simulink model "Refined_Model_39"  (R2020b)
settings: Solver=FixedStepAuto  StartTime=0.0  StopTime=300  FixedStep=dt  RelTol=1e-3
values from neighbouring files (symbols this model uses):
  ALInpSpeed = AxlLoss (1,:)    [GPS_val.m]    (also in ICEBEV_Script.m; ICEBEV_Script_VECTO.m; ICE_Script.m; ICE_Script_SSVal.m)
  ALInpTor = AxlLoss(:,1)    [GPS_val.m]    (also in ICEBEV_Script.m; ICEBEV_Script_VECTO.m; ICE_Script.m; ICE_Script_SSVal.m)
  ALTableVal = AxlLoss(2:end,2:end)    [GPS_val.m]    (also in ICEBEV_Script.m; ICEBEV_Script_VECTO.m; ICE_Script.m; ICE_Script_SSVal.m)
  CovDist = RoadProfile(:,4)    [ICE_Val.m]
  Cx = VehicleDefine(7,3)    [BEV_Basictest.m]    (also in GPS_val.m; ICEBEV_Script.m; ICEBEV_Script_VECTO.m; ICE_Script.m)
  Dist = 1:length(MaxSpeedProfile)    [GPS_val.m]    (also in ICE_Script.m; ICE_Val.m = [1:CovDist(end)])
  DynRolRad = VehicleDefine(5,3)    [BEV_Basictest.m]    (also in GPS_val.m; ICEBEV_Script.m; ICEBEV_Script_VECTO.m; ICE_Script.m)
  EngineRpm = round(IntpTorCur(:,1))    [GPS_val.m]    (also in ICEBEV_Script.m; ICEBEV_Script_VECTO.m; ICE_Script.m; ICE_Script_SSVal.m)
  EngineRpmUse = [EngineRpmUse1; EngineRpmUse2]    [GPS_val.m]    (also in ICEBEV_Script.m; ICEBEV_Script_VECTO.m; ICE_Script.m; ICE_Script_SSVal.m)
  etaClutch = VehicleDefine(23,3)    [GPS_val.m]    (also in ICEBEV_Script.m; ICEBEV_Script_VECTO.m; ICE_Script.m; ICE_Script_SSVal.m)
  FCTableVal = FCMap(2:end,2:end)    [GPS_val.m]    (also in ICEBEV_Script.m; ICEBEV_Script_VECTO.m; ICE_Script.m; ICE_Script_SSVal.m)
  FDR = VehicleDefine(20,3)    [BEV_Basictest.m]    (also in GPS_val.m = VehicleDefine(22,3); ICEBEV_Script.m = VehicleDefine(22,3); ICEBEV_Script_VECTO.m = VehicleDefine(22,3); ICE_Script.m = VehicleDefine(22,3))
  Fr = VehicleDefine(13,3)    [BEV_Basictest.m]    (also in GPS_val.m; ICEBEV_Script.m; ICEBEV_Script_VECTO.m; ICE_Script.m)
  g = VehicleDefine(14,3)    [BEV_Basictest.m]    (also in GPS_val.m; ICEBEV_Script.m; ICEBEV_Script_VECTO.m; ICE_Script.m)
  GNo = GBXDefine(:,1)    [GPS_val.m]    (also in ICEBEV_Script.m; ICEBEV_Script_VECTO.m; ICE_Script.m; ICE_Script_SSVal.m)
  GRa = GBXDefine(:,2)    [GPS_val.m]    (also in ICEBEV_Script.m; ICEBEV_Script_VECTO.m; ICE_Script.m; ICE_Script_SSVal.m)
  InitVel = VehicleDefine(21,3)    [BEV_Basictest.m]    (also in GPS_val.m = VehicleDefine(24,3); ICEBEV_Script.m = VehicleDefine(24,3); ICEBEV_Script_VECTO.m = VehicleDefine(24,3); ICE_Script.m = VehicleDefine(24,3))
  IntpSlope = round(IntpSlope,1)    [GPS_val.m]    (also in ICE_Script.m; ICE_Val.m = A)
  Je = VehicleDefine(25,3)    [GPS_val.m]    (also in ICEBEV_Script.m; ICEBEV_Script_VECTO.m; ICE_Script.m; ICE_Script_SSVal.m)
  Jk = VehicleDefine(15,3)    [BEV_Basictest.m]    (also in GPS_val.m; ICEBEV_Script.m; ICEBEV_Script_VECTO.m; ICE_Script.m)
  Jm = VehicleDefine(16,3)    [GPS_val.m]    (also in ICEBEV_Script.m; ICEBEV_Script_VECTO.m; ICE_Script.m; ICE_Script_SSVal.m)
  MaxAcc = 1    [BEV_Basictest.m]    (also in GPS_val.m; ICEBEV_Script.m; ICEBEV_Script_VECTO.m; ICE_Script.m)
  MaxDec = 1    [BEV_Basictest.m]    (also in GPS_val.m; ICEBEV_Script.m; ICEBEV_Script_VECTO.m; ICE_Script.m)
  MaxSpeedProfile = FMSP    [GPS_val.m]    (also in ICE_Script.m; ICE_Val.m = repelem(SegSPLatinmps,SegLeninm))
  MaxTorValThrot = max(ThrotTableVal,[],2)    [GPS_val.m]    (also in ICEBEV_Script.m; ICEBEV_Script_VECTO.m; ICE_Script.m; ICE_Script_SSVal.m)
  Me = VehicleDefine(10,3)    [BEV_Basictest.m]    (also in GPS_val.m; ICEBEV_Script.m; ICEBEV_Script_VECTO.m; ICE_Script.m)
  MotoringTor = IntpTorCur(:,3)    [GPS_val.m]    (also in ICEBEV_Script.m; ICEBEV_Script_VECTO.m; ICE_Script.m; ICE_Script_SSVal.m)
  Mt = VehicleDefine(12,3)    [BEV_Basictest.m]    (also in GPS_val.m; ICEBEV_Script.m; ICEBEV_Script_VECTO.m; ICE_Script.m)
  Mtot = Mv+Me+Mt    [BEV_Basictest.m]    (also in GPS_val.m; ICEBEV_Script.m; ICEBEV_Script_VECTO.m; ICE_Script.m)
  Mv = VehicleDefine(9,3)    [BEV_Basictest.m]    (also in GPS_val.m; ICEBEV_Script.m; ICEBEV_Script_VECTO.m; ICE_Script.m)
  NoSteps = round(Dist(end))    [GPS_val.m]    (also in ICE_Script.m; ICE_Val.m = 3002)
  NoWhlFA = VehicleDefine(2,3)    [BEV_Basictest.m]    (also in GPS_val.m; ICE_Script.m; ICE_Val.m; ICE_Val_new.m)
  NoWhlRA = VehicleDefine(4,3)    [BEV_Basictest.m]    (also in GPS_val.m; ICE_Script.m; ICE_Val.m; ICE_Val_new.m)
  rho = VehicleDefine(6,3)    [BEV_Basictest.m]    (also in GPS_val.m; ICEBEV_Script.m; ICEBEV_Script_VECTO.m; ICE_Script.m)
  RpmBrkPnt = ThrottleMap(1,:)    [GPS_val.m]    (also in ICEBEV_Script.m; ICEBEV_Script_VECTO.m; ICE_Script.m; ICE_Script_SSVal.m)
  s = divisors(length(MaxSpeedProfile))    [GPS_val.m]    (also in ICEBEV_Script.m = round(FLoadTor); ICEBEV_Script_VECTO.m = round(FLoadTor); ICE_Script.m = round(FLoadTor); ICE_Script_SSVal.m = round(FLoadTor))
  SegNo = RoadProfile(:,1)    [ICE_Val.m]
  SegSPLatinmps = (sqrt(aMaxLat*g*CurRadinm))    [GPS_val.m]    (also in ICE_Script.m; ICE_Val.m)
  Sx = VehicleDefine(8,3)    [BEV_Basictest.m]    (also in GPS_val.m; ICEBEV_Script.m; ICEBEV_Script_VECTO.m; ICE_Script.m)
  ThrotPos = ThrotPos'    [GPS_val.m]    (also in ICEBEV_Script.m; ICEBEV_Script_VECTO.m; ICE_Script.m; ICE_Script_SSVal.m)
  ThrotTableVal = ThrottleMap(2:end,2:end)    [GPS_val.m]    (also in ICEBEV_Script.m; ICEBEV_Script_VECTO.m; ICE_Script.m; ICE_Script_SSVal.m)
undefined symbols (not defined in the file or in its folder): G1Inprpm, GInprpm, GInpTor, Gmot, GTorLoss, Jgbx, MaxSpinG, MaxWhlTorinG, Stoptimes
libraries: simulink x4, autolibshared x2, vehdynlibtire x2, autolibdatasheetbattery x1, autolibmappedmotor x1
(part 3 of 4)

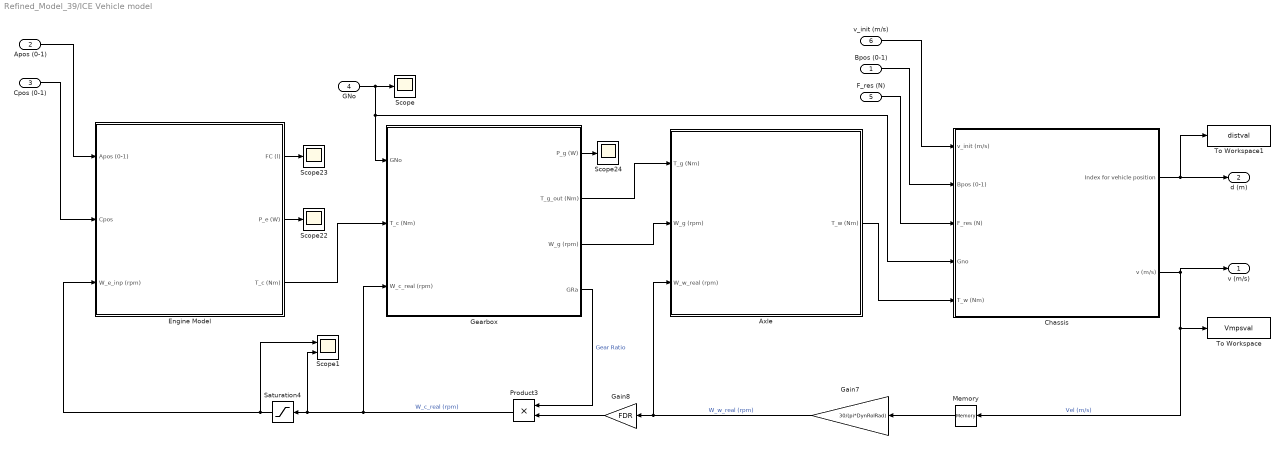
== system Refined_Model_39/ICE Vehicle model ==
  Bpos (0-1) : Inport
  Apos (0-1) : Inport  Port=2
  Cpos (0-1) : Inport  Port=3
  GNo : Inport  Port=4
  F_res (N) : Inport  Port=5
  v_init (m/s) : Inport  Port=6
  Axle : Subsystem
  Chassis : Subsystem
  Engine Model : Subsystem
  Gain7 : Gain  Gain=30/(pi*DynRolRad)
  Gain8 : Gain  Gain=FDR
  Gearbox : Subsystem
  Memory : Memory
  Product3 : Product
  Saturation4 : Saturate  UpperLimit=max(EngineRpmUse)  LowerLimit=min(EngineRpmUse)
  Scope{,22..24} (4 alike) : Scope
  Scope1 : Scope  NumInputPorts=2
  To Workspace : ToWorkspace  VariableName=Vmpsval  SaveFormat=Timeseries  SampleTime=-1
  To Workspace1 : ToWorkspace  VariableName=distval  SaveFormat=Timeseries  SampleTime=-1
  v (m/s) : Outport
  d (m) : Outport  Port=2
  wires:
  Gearbox/2(T_g_out (Nm)) -> Axle/1(T_g (Nm))
  Gearbox/3(W_g (rpm)) -> Axle/2(W_g (rpm))
  Chassis/1(Index for vehicle position) -> To Workspace1/1, d (m)/1
  Bpos (0-1)/1 -> Chassis/2(Bpos (0-1))
  v_init (m/s)/1 -> Chassis/1(v_init (m/s))
  Axle/1(T_w (Nm)) -> Chassis/5(T_w (Nm))
  F_res (N)/1 -> Chassis/3(F_res (N))
  Gearbox/1(P_g (W)) -> Scope24/1
  Engine Model/3(T_c (Nm)) -> Gearbox/2(T_c (Nm))
  Apos (0-1)/1 -> Engine Model/1(Apos (0-1))
  Engine Model/2(P_e (W)) -> Scope22/1
  Engine Model/1(FC (l)) -> Scope23/1
  GNo/1 -> Chassis/4(Gno), Gearbox/1(GNo), Scope/1
  Chassis/2(v (m/s)) -> v (m/s)/1, Memory/1, To Workspace/1  "Vel (m/s)"
  Gearbox/4(GRa) -> Product3/1  "Gear Ratio"
  Gain8/1 -> Product3/2
  Gain7/1 -> Gain8/1, Axle/3(W_w_real (rpm))  "W_w_real (rpm)"
  Cpos (0-1)/1 -> Engine Model/2(Cpos)
  Product3/1 -> Scope1/2, Saturation4/1, Gearbox/3(W_c_real (rpm))  "W_c_real (rpm)"
  Saturation4/1 -> Scope1/1, Engine Model/3(W_e_inp (rpm))
  Memory/1 -> Gain7/1

== system Refined_Model_39/BEV model/Axle ==
  T_g (Nm) : Inport
  W_g (rpm) : Inport  Port=2
  W_w_real (rpm) : Inport  Port=3
  Add4 : Sum  Inputs=-++
  Add5 : Sum
  Axle Loss Tables1 : Lookup_n-D  BreakpointsForDimension1=ALInpTor  BreakpointsForDimension2=ALInpSpeed  BreakpointsForDimension3=GNo  Table=ALTableVal  InterpMethod=Linear Lagrange  InternalRulePriority=Speed  RndMeth=Simplest  InputSameDT=on
      settings: InputPortMap=u0,u1
  Constant28 : Constant  Value=NoWhlFA
  Constant29 : Constant  Value=NoWhlRA
  Derivative6 : Derivative
  FDR4 : Gain  Gain=FDR
  FDR5 : Gain  Gain=1/FDR
  Gain12 : Gain  Gain=pi/30
  Product10 : Product
  Scope : Scope
  Scope2 : Scope  NumInputPorts=2
  Wheel Inertia : Gain  Gain=Jk
  T_w (Nm) : Outport
  wires:
  Product10/1 -> Add4/3  "T_w_iner (Nm)"
  Derivative6/1 -> Wheel Inertia/1
  Add5/1 -> Product10/2
  Constant29/1 -> Add5/2
  Constant28/1 -> Add5/1
  FDR4/1 -> Add4/2
  FDR5/1 -> Scope2/2  "W_w (rpm)"
  Wheel Inertia/1 -> Product10/1
  Add4/1 -> T_w (Nm)/1, Scope/1  "T_w (Nm)"
  T_g (Nm)/1 -> Axle Loss Tables1/1, FDR4/1
  W_g (rpm)/1 -> FDR5/1
  W_w_real (rpm)/1 -> Gain12/1
  Axle Loss Tables1/1 -> Add4/1  "T_axl_loss (Nm)"
  Gain12/1 -> Scope2/1, Axle Loss Tables1/2, Derivative6/1

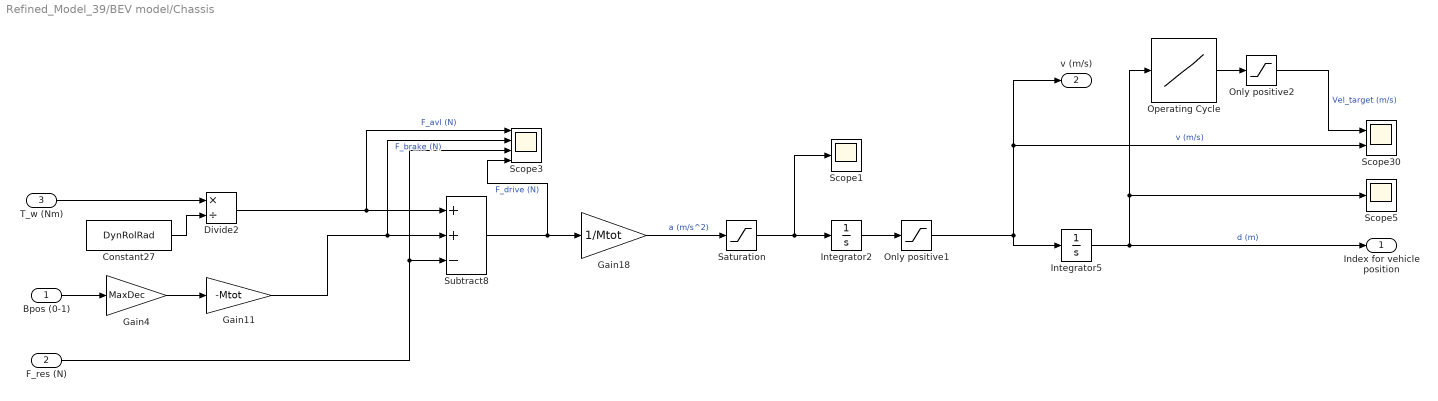
== system Refined_Model_39/BEV model/Chassis ==
  Bpos (0-1) : Inport
  F_res (N) : Inport  Port=2
  T_w (Nm) : Inport  Port=3
  Constant27 : Constant  Value=DynRolRad
  Divide2 : Product  Inputs=*/
  Gain11 : Gain  Gain=-Mtot
  Gain18 : Gain  Gain=1/Mtot
  Gain4 : Gain  Gain=MaxDec
  Integrator2 : Integrator  ContinuousStateAttributes='acceleration'
  Integrator5 : Integrator  ContinuousStateAttributes='velocity'
  Only positive1 : Saturate  UpperLimit=inf  LowerLimit=0
  Only positive2 : Saturate  UpperLimit=inf  LowerLimit=0
  Operating Cycle : Lookup_n-D  NumberOfTableDimensions=1  BreakpointsForDimension1=Dist  BreakpointsForDimension2=G1Inprpm  Table=MaxSpeedProfile  InterpMethod=Linear Lagrange  InternalRulePriority=Speed  RndMeth=Simplest  InputSameDT=on
  Saturation : Saturate  UpperLimit=MaxAcc  LowerLimit=-(MaxDec)
  Scope1 : Scope
  Scope3 : Scope  NumInputPorts=4
  Scope30 : Scope  NumInputPorts=2
  Scope5 : Scope
  Subtract8 : Sum  Inputs=++-
  Index for vehicle position : Outport
  v (m/s) : Outport  Port=2
  wires:
  Constant27/1 -> Divide2/2
  Subtract8/1 -> Scope3/4, Gain18/1  "F_drive (N)"
  Divide2/1 -> Subtract8/1, Scope3/1  "F_avl (N)"
  Integrator5/1 -> Index for vehicle position/1, Scope5/1, Operating Cycle/1  "d (m)"
  Integrator2/1 -> Only positive1/1
  T_w (Nm)/1 -> Divide2/1
  Gain11/1 -> Subtract8/2, Scope3/2  "F_brake (N)"
  Only positive1/1 -> v (m/s)/1, Scope30/2, Integrator5/1  "v (m/s)"
  Operating Cycle/1 -> Only positive2/1
  Gain18/1 -> Saturation/1  "a (m/s^2)"
  Bpos (0-1)/1 -> Gain4/1
  Gain4/1 -> Gain11/1
  F_res (N)/1 -> Subtract8/3, Scope3/3
  Saturation/1 -> Integrator2/1, Scope1/1
  Only positive2/1 -> Scope30/1  "Vel_target (m/s)"

== system Refined_Model_39/BEV model/Electric Powertrain ==
  TrqCmd : Inport
  W_m (rpm) : Inport  Port=2
  Add : Sum
  Ambient Temperature : Constant  Value=27
  Datasheet Battery : autolibdatasheetbattery/Datasheet Battery  CapacityCtrl=Parameter  OutputVlt=Unfiltered  BattChargeMax=100  Em=[2.8 3.228 3.284 3.361 3.408 3.427 3.472 3.477 3.493 3.504 3.516 3.528 3.537 3.545 3.555 3.561 3.566 3.576 3.587 3.589 3.594 3.6 3.608 3.61 3.616 3.619 3.626 3.632 3.637 3.64 3.645 3.646 3.652 3.655 3.658 3.661 3.664 3.668 3.673 3.678 3.68 3.681 3.686 3.692 3.699 3.702 3.705 3.71 3.717 3.723 3.728 3.733 3.735 3.742 3.749 3.755 3.761 3.768 3.773 3.78 3.791 3.798 3.798 3.814 3.818 3.825 3.841 3.846 3.855 3.863 3.877 3.885 3.894 3.907 3.919 3.926 3.935 3.944 3.954 3.964 3.974 3.988 3.998 4.014 4.029 4.034 4.047 4.065 4.074 4.086 4.097 4.131 4.126 4.138 4.15 4.18 4.174 4.187 4.207 4.231 4.221]  CapLUTBp=[0 0.01 0.02 0.03 0.04 0.05 0.06 0.07 0.08 0.09 0.1 0.11 0.12 0.13 0.14 0.15 0.16 0.17 0.18 0.19 0.2 0.21 0.22 0.23 0.24 0.25 0.26 0.27 0.28 0.29 0.3 0.31 0.32 0.33 0.34 0.35 0.36 0.37 0.38 0.39 0.4 0.41 0.42 0.43 0.44 0.45 0.46 0.47 0.48 0.49 0.5 0.51 0.52 0.53 0.54 0.55 0.56 0.57 0.58 0.59 0.6 0.61 0.62 0.63 0.64 0.65 0.66 0.67 0.68 0.69 0.7 0.71 0.72 0.73 0.74 0.75 0.76 0.77 0.78 0.79 0.8 0.81 0.82 0.83 0.84 0.85 0.86 0.87 0.88 0.89 0.9 0.91 0.92 0.93 0.94 0.95 0.96 0.97 0.98 0.99 1]  RInt=[0.008846 0.009319 0.009027 0.00847 0.01032 0.01314;0.006389 0.006554 0.005553 0.005525 0.006043 0.007805;0.004364 0.004101 0.00406 0.003452 0.003846 0.004517;0.002031 0.002563 0.002532 0.00246 0.002716 0.003047;0.001443 0.001825 0.001795 0.001778 0.001924 0.002234;0.0005603 0.0007192 0.0006887 0.0007557 0.0007355 0.001014;0.001028 0.001338 0.001 0.001536 0.001546 0.002789]  BattTempBp=[243.1 253.1 263.1 273.1 283.1 298.1 313.1]  CapSOCBp=[0 0.2 0.4 0.6 0.8 1]  Ns=1  Np=1  BattCapInit=100  Tc=1/1000  Vinit=4.221  RefBlkName='autolibdatasheetbattery/Datasheet Battery'
      settings: SourceProductBaseCode=PW
  Gain12 : Gain  Gain=pi/30
  Mapped Motor : autolibmappedmotor/Mapped Motor  port_config=Speed  param_by=Tabulated torque-speed envelope  w_t=[ 0 375 750 800 ]  T_t=[0.09 0.08 0.07 0]  torque_max=.1  power_max=30  Tc=0.02  param_loss=Single efficiency measurement  eff=100  w_eff=375  T_eff=0.08  Piron=0  Pbase=0  w_eff_bp=[-8000 -4000 0 4000 8000]  T_eff_bp=[0 0.03 0.06 0.09]  Temp_eff_bp=[233.15 293.15 373.15]  losses_table=[1.49 1.67 2.21 3.10; 0.42 0.69 1.14 2.03; 0.06 0.24 0.78 1.68; 0.42 0.69 1.14 2.03; 1.49 1.67 2.21 3.10]  losses_table_3d=cat(3,1.05*[1.49 1.67 2.21 3.10; 0.42 0.69 1.14 2.03; 0.06 0.24 0.78 1.68; 0.42 0.69 1.14 2.03; 1.49 1.67 2.21 3.10],[1.49 1.67 2.21 3.10; 0.42 0.69 1.14 2.03; 0.06 0.24 0.78 1.68; 0.42 0.69 1.14 2.03; 1.49 1.67 2.21 3.10],1.03*[1.49 1.67 2.21 3.10; 0.42 0.69 1.14 2.03; 0.06 0.24 0.78 1.68; 0.42 0.69 1.14 2.03; 1.49 1.67 2.21 3.10])  efficiency_table=[95 95 95 95; 95 95 95 95; 95 95 95 95; 95 95 95 95; 95 95 95 95]  efficiency_table_3d=cat(3,90*ones(5,4),95*ones(5,4),92*ones(5,4))  J=5e-6  b=1e-5  omega_o=0  T_t_extended=[0 0.07 0.08 0.09 0.08 0.07 0]  w_t_extended=[-800 -750 -375 0 375 750 800]  KLossIron=0  KLossCopper=0  x_w_eff_vec=[-8000 -4000 0 4000 8000]  x_T_eff_vec=[-0.09 -0.06 -0.03 0 0.03 0.06 0.09]  x_tmp_eff_vec=[233.15 293.15 373.15]  x_losses_mat=[3.1 2.21 1.67 1.49 1.67 2.21 3.1;2.03 1.14 0.69 0.42 0.69 1.14 2.03;1.68 0.78 0.24 0.06 0.24 0.78 1.68;2.03 1.14 0.69 0.42 0.69 1.14 2.03;3.1 2.21 1.67 1.49 1.67 2.21 3.1]  x_losses_mat_3d=cat(3,[3.255 2.3205 1.7535 1.5645 1.7535 2.3205 3.255;2.1315 1.197 0.7245 0.441 0.7245 1.197 2.1315;1.764 0.819 0.252 0.063 0.252 0.819 1.764;2.1315 1.197 0.7245 0.441 0.7245 1.197 2.1315;3.255 2.3205 1.7535 1.5645 1.7535 2.3205 3.255],[3.1 2.21 1.67 1.49 1.67 2.21 3.1;2.03 1.14 0.69 0.42 0.69 1.14 2.03;1.68 0.78 0.24 0.06 0.24 0.78 1.68;2.03 1.14 0.69 0.42 0.69 1.14 2.03;3.1 2.21 1.67 1.49 1.67 2.21 3.1],[3.193 2.2763 1.7201 1.5347 1.7201 2.2763 3.193;2.0909 1.1742 0.7107 0.4326 0.7107 1.1742 2.0909;1.7304 0.8034 0.2472 0.0618 0.2472 0.8034 1.7304;2.0909 1.1742 0.7107 0.4326 0.7107 1.1742 2.0909;3.193 2.2763 1.7201 1.5347 1.7201 2.2763 3.193])  CalLossMapData={}  CalLossWithTempMapData={}  aMode=2  RefBlkName='autolibmappedmotor/Mapped Motor'
      settings: SourceProductBaseCode=PW,MT,UV,VE,VP
  Terminator : Terminator
  Terminator1 : Terminator
  to Kelvin : Constant  Value=273
  MtrTrq : Outport
  wires:
  Mapped Motor/3 -> MtrTrq/1
  Ambient Temperature/1 -> Add/1
  Datasheet Battery/2 -> Mapped Motor/1  "BattVolt[V]"
  W_m (rpm)/1 -> Gain12/1
  Mapped Motor/2 -> Datasheet Battery/1  "BattCurr[A]"
  to Kelvin/1 -> Add/2
  Add/1 -> Datasheet Battery/2
  TrqCmd/1 -> Mapped Motor/3
  Gain12/1 -> Mapped Motor/2  "W_m (rad/s)"
  Datasheet Battery/1 -> Terminator/1
  Mapped Motor/1 -> Terminator1/1

== system Refined_Model_39/BEV model/Motor Gearbox ==
  T_m (Nm) : Inport
  W_m_ real (rpm) : Inport  Port=2
  Add1 : Sum
  Derivative5 : Derivative
  Divide : Product  Inputs=*/
  Gain : Gain  Gain=30/pi
  Gain12 : Gain  Gain=pi/30
  Gain17 : Gain  Gain=Jgbx
  Motor gbx ratio : Constant  Value=Gmot
  Product7 : Product
  T_m_out (Nm) : Outport
  W_m (rpm) : Outport  Port=2
  wires:
  Motor gbx ratio/1 -> Product7/2, Divide/2
  Divide/1 -> Gain/1
  Gain/1 -> W_m (rpm)/1
  W_m_ real (rpm)/1 -> Divide/1, Gain12/1
  Add1/1 -> Product7/1
  Derivative5/1 -> Gain17/1  "W_m_dot (rad/s^2)"
  Gain17/1 -> Add1/2
  Product7/1 -> T_m_out (Nm)/1  "T_m_out (Nm)"
  T_m (Nm)/1 -> Add1/1
  Gain12/1 -> Derivative5/1

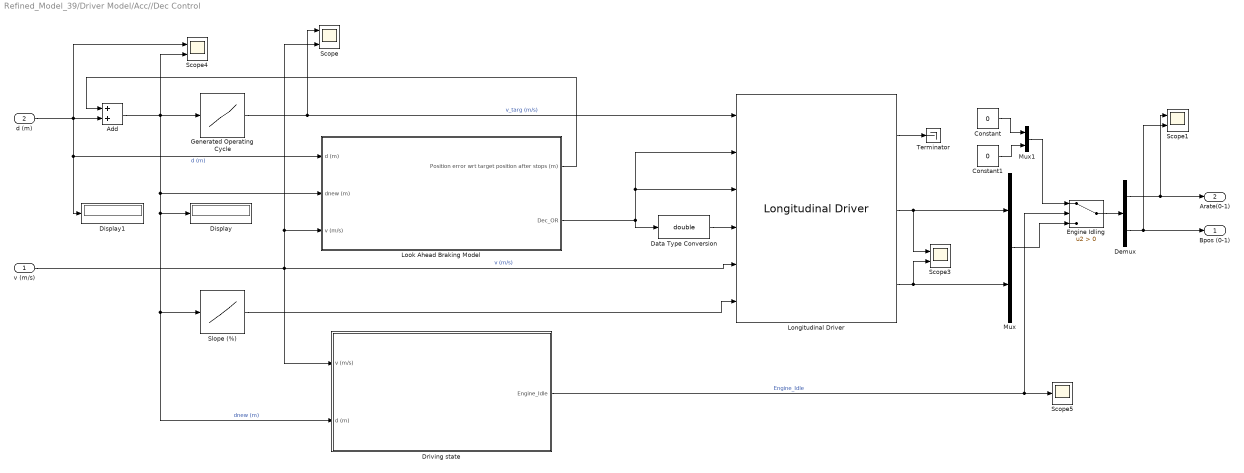
== system Refined_Model_39/Driver Model/Acc//Dec Control ==
  v (m/s) : Inport
  d (m) : Inport  Port=2
  Add : Sum
  Constant : Constant  Value=0
  Constant1 : Constant  Value=0
  Data Type Conversion : DataTypeConversion  OutDataTypeStr=double
  Demux : Demux  Outputs=2
  Display : Display
  Display1 : Display
  Driving state : Subsystem
  Engine Idling : Switch  Criteria=u2 > Threshold
  Generated Operating Cycle : Lookup_n-D  NumberOfTableDimensions=1  BreakpointsForDimension1=Dist  BreakpointsForDimension2=G1Inprpm  Table=MaxSpeedProfile  InterpMethod=Linear Lagrange  InternalRulePriority=Speed  RndMeth=Simplest  InputSameDT=on
  Longitudinal Driver : autolibshared/Longitudinal Driver  extAccelOvr=off  extDecelOvr=on  extAccelHld=off  extDecelHld=off  extAccelZero=on  extDecelZero=off  cntrlType=PI  shftType=None  velUnits=m/s  gearOut=off  Kp=200  Ki=150  Kff=0  Kg=0  VehVelVec=[0 100]  KffVec=[.1 .1]  KpVec=[10 10]  KiVec=[5 5]  KgVec=[0 0]  m=1500  Kpt=3000  tau=.1  L=2  aR=200  bR=2.5  cR=.5  g=9.81  vnom=100  Kaw=0  tauerr=0  tauPt=2  GearInit=0  tShift=.1  pdlVec=[0.1 0.4 0.5 0.9]  upShftTbl=[-1 12.9375 26.4375 39.9375 51.18749999999999 62.4375 72.84375 83.25;-1 16.3125 29.8125 43.3125 54.5624 65.8125 76.78125 87.75;-1 19.6875 33.1875 46.68749999999999 57.9375 69.1875 80.71875 92.25;-1 33 52.5 77.25 100.5 138.75 161.875 185]  dwnShftTbl=[1 9.5625 23.0625 36.5625 47.8125 59.0625 68.90625 78.75;1 12.9375 26.4375 39.9375 51.18749999999999 62.4375 72.84375 83.25;1 16.3125 29.8125 43.3125 54.562499 65.8125 76.78125 87.75;1 19.6875 33.1875 46.68749999999999 57.9375 69.1875 80.71875 92.25]  tClutch=.5  tRev=.5  tPark=120  aMode=1  UpGearVec="[0  1  2  3  4  5  6  7]"  DownGearVec="[1  2  3  4  5  6  7  8]"
      settings: SourceProductBaseCode=PW,MT,UV,VE,VP
  Look Ahead Braking Model : Subsystem
  Mux : Mux  Inputs=2
  Mux1 : Mux  Inputs=2
  Scope : Scope  NumInputPorts=3
  Scope1 : Scope  NumInputPorts=2
  Scope3 : Scope  NumInputPorts=2
  Scope4 : Scope  NumInputPorts=2
  Scope5 : Scope
  Slope (%) : Lookup_n-D  NumberOfTableDimensions=1  BreakpointsForDimension1=Dist  Table=IntpSlope  InternalRulePriority=Speed  RndMeth=Simplest  InputSameDT=on
  Terminator : Terminator
  Bpos (0-1) : Outport
  Arate(0-1) : Outport  Port=2
  wires:
  Slope (%)/1 -> Longitudinal Driver/6
  Demux/1 -> Scope1/1, Arate(0-1)/1
  Demux/2 -> Bpos (0-1)/1, Scope1/2
  Constant/1 -> Mux1/1
  Mux/1 -> Engine Idling/3
  Constant1/1 -> Mux1/2
  Mux1/1 -> Engine Idling/1
  Engine Idling/1 -> Demux/1
  Add/1 -> Generated Operating Cycle/1, Scope4/2, Display/1, Driving state/2(d (m)), Slope (%)/1, Look Ahead Braking Model/2(dnew (m))  "dnew (m)"
  v (m/s)/1 -> Driving state/1(v (m/s)), Scope/3, Look Ahead Braking Model/3(v (m/s)), Longitudinal Driver/5  "v (m/s)"
  Generated Operating Cycle/1 -> Scope/1, Longitudinal Driver/1  "v_targ (m/s)"
  Data Type Conversion/1 -> Longitudinal Driver/4
  Longitudinal Driver/3 -> Mux/2, Scope3/2
  Driving state/1(Engine_Idle) -> Scope5/1, Engine Idling/2  "Engine_Idle"
  Look Ahead Braking Model/2(Dec_OR) -> Longitudinal Driver/2, Longitudinal Driver/3, Data Type Conversion/1
  Longitudinal Driver/2 -> Mux/1, Scope3/1
  d (m)/1 -> Scope4/1, Look Ahead Braking Model/1(d (m)), Display1/1, Add/2  "d (m)"
  Look Ahead Braking Model/1(Position error wrt target position after stops (m)) -> Add/1
  Longitudinal Driver/1 -> Terminator/1

== system Refined_Model_39/Driver Model/Driver Throttle Mapping BEV ==
  F_res (N) : Inport
  Arate(0-1) : Inport  Port=2
  Add : Sum
  Gain1 : Gain  Gain=MaxAcc
  Gain10 : Gain  Gain=1/FDR
  Gain3 : Gain  Gain=1/Gmot
  Gain4 : Gain  Gain=Mtot
  Gain9 : Gain  Gain=DynRolRad
  T_req (Nm) : Outport
  wires:
  Gain3/1 -> T_req (Nm)/1  "T_req (Nm)"
  Gain1/1 -> Gain4/1
  Gain9/1 -> Gain10/1
  Add/1 -> Gain9/1  "T_w_req (Nm)"
  Gain4/1 -> Add/2
  Gain10/1 -> Gain3/1
  F_res (N)/1 -> Add/1
  Arate(0-1)/1 -> Gain1/1

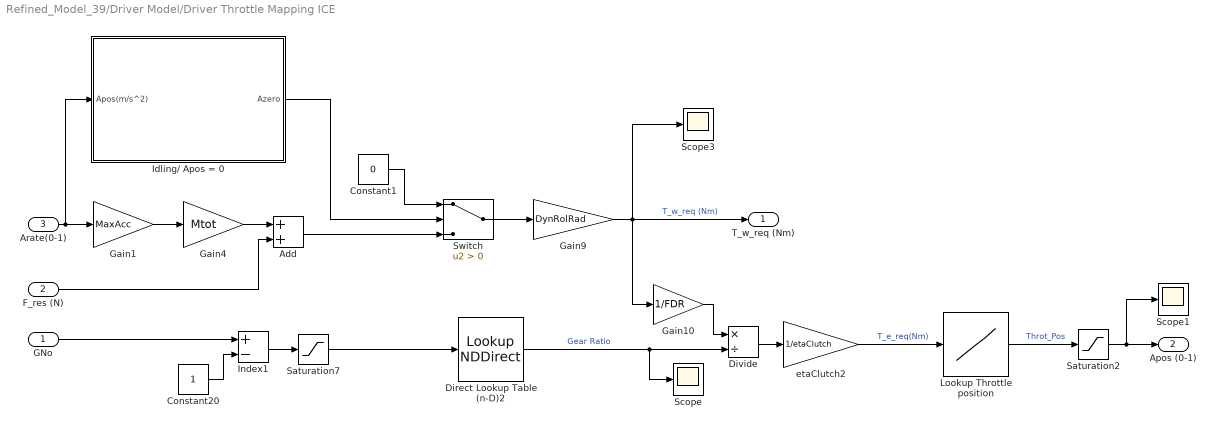
== system Refined_Model_39/Driver Model/Driver Throttle Mapping ICE ==
  GNo : Inport
  F_res (N) : Inport  Port=2
  Arate(0-1) : Inport  Port=3
  Add : Sum
  Constant1 : Constant  Value=0
  Constant20 : Constant
  Direct Lookup Table (n-D)2 : LookupNDDirect  NumberOfTableDimensions=1  Table=GRa
  Divide : Product  Inputs=*/
  Gain1 : Gain  Gain=MaxAcc
  Gain10 : Gain  Gain=1/FDR
  Gain4 : Gain  Gain=Mtot
  Gain9 : Gain  Gain=DynRolRad
  Idling/ Apos = 0 : Subsystem
  Index1 : Sum  Inputs=+-
  Lookup Throttle position : Lookup_n-D  NumberOfTableDimensions=1  BreakpointsForDimension1=MaxTorValThrot  Table=ThrotPos  InternalRulePriority=Speed  RndMeth=Simplest  InputSameDT=on
  Saturation2 : Saturate  UpperLimit=1  LowerLimit=0
  Saturation7 : Saturate  UpperLimit=inf  LowerLimit=0
  Scope : Scope
  Scope1 : Scope
  Scope3 : Scope
  Switch : Switch  Criteria=u2 > Threshold
  etaClutch2 : Gain  Gain=1/etaClutch
  T_w_req (Nm) : Outport
  Apos (0-1) : Outport  Port=2
  wires:
  etaClutch2/1 -> Lookup Throttle position/1  "T_e_req(Nm)"
  Add/1 -> Switch/3
  Gain9/1 -> Scope3/1, T_w_req (Nm)/1, Gain10/1  "T_w_req (Nm)"
  Gain10/1 -> Divide/1
  Gain4/1 -> Add/1
  Divide/1 -> etaClutch2/1
  F_res (N)/1 -> Add/2
  Lookup Throttle position/1 -> Saturation2/1  "Throt_Pos"
  Saturation2/1 -> Apos (0-1)/1, Scope1/1
  Arate(0-1)/1 -> Idling/ Apos = 0/1(Apos(m/s^2)), Gain1/1
  Gain1/1 -> Gain4/1
  Constant20/1 -> Index1/2
  GNo/1 -> Index1/1
  Index1/1 -> Saturation7/1
  Saturation7/1 -> Direct Lookup Table (n-D)2/1
  Direct Lookup Table (n-D)2/1 -> Scope/1, Divide/2  "Gear Ratio"
  Switch/1 -> Gain9/1
  Constant1/1 -> Switch/1
  Idling/ Apos = 0/1(Azero) -> Switch/2

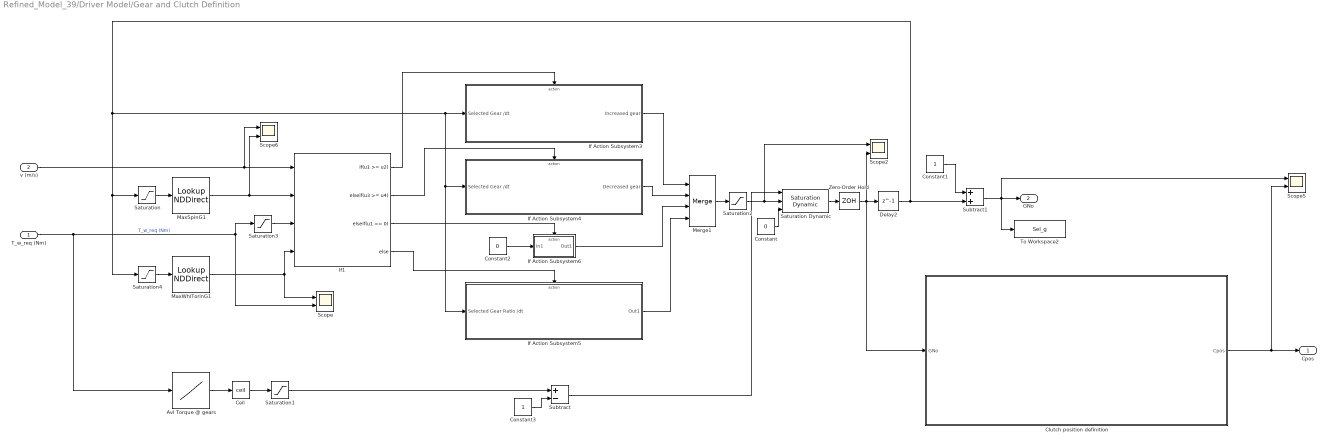
== system Refined_Model_39/Driver Model/Gear and Clutch Definition ==
  T_w_req (Nm) : Inport
  v (m/s) : Inport  Port=2
  Avl Torque @ gears : Lookup_n-D  NumberOfTableDimensions=1  BreakpointsForDimension1=flip(MaxWhlTorinG)  Table=flip(GNo)  InternalRulePriority=Speed  RndMeth=Simplest  InputSameDT=on
  Ceil : Rounding  Operator=ceil
  Clutch position definition : Subsystem
  Constant : Constant  Value=0
  Constant1 : Constant
  Constant2 : Constant  Value=0
  Constant3 : Constant
  Delay2 : Delay  DelayLength=1
  If Action Subsystem3 : Subsystem  TreatAsAtomicUnit=on
  If Action Subsystem4 : Subsystem  TreatAsAtomicUnit=on
  If Action Subsystem5 : Subsystem  TreatAsAtomicUnit=on
  If Action Subsystem6 : Subsystem  TreatAsAtomicUnit=on
  If1 : If  NumInputs=4  IfExpression=u1 >= u2  ElseIfExpressions=u3 >= u4,u1 == 0
  MaxSpinG1 : LookupNDDirect  NumberOfTableDimensions=1  Table=MaxSpinG
  MaxWhlTorinG1 : LookupNDDirect  NumberOfTableDimensions=1  Table=MaxWhlTorinG
  Merge1 : Merge  Inputs=4
  Saturation : Saturate  UpperLimit=inf  LowerLimit=0
  Saturation Dynamic : simulink/Discontinuities/Saturation Dynamic  OutMin=[]  OutMax=[]  OutDataTypeStr=Inherit: Same as second input  OutDataType=fixdt(1, 16)  OutScaling=2^-10  DoSatur=off
  Saturation1 : Saturate  UpperLimit=max(GNo)  LowerLimit=0
  Saturation2 : Saturate  UpperLimit=max(GNo)-1  LowerLimit=0
  Saturation3 : Saturate  UpperLimit=inf  LowerLimit=0
  Saturation4 : Saturate  UpperLimit=inf  LowerLimit=0
  Scope{,2,5..6} (4 alike) : Scope  NumInputPorts=2
  Subtract : Sum  Inputs=+-
  Subtract1 : Sum
  To Workspace2 : ToWorkspace  VariableName=Sel_g  SaveFormat=Timeseries  SampleTime=-1
  Zero-Order Hold : ZeroOrderHold  SampleTime=3
  Cpos : Outport
  GNo : Outport  Port=2
  wires:
  Clutch position definition/1(Cpos) -> Scope5/2, Cpos/1
  If1/2 -> If Action Subsystem4/Action
  If Action Subsystem4/1(Decreased gear) -> Merge1/2
  If1/4 -> If Action Subsystem5/Action
  If Action Subsystem3/1(Increased gear) -> Merge1/1
  MaxSpinG1/1 -> Scope6/2, If1/2
  If Action Subsystem5/1(Out1) -> Merge1/4
  MaxWhlTorinG1/1 -> Scope/1, If1/4
  If1/1 -> If Action Subsystem3/Action
  Saturation3/1 -> If1/3
  T_w_req (Nm)/1 -> Saturation3/1, Scope/2, Avl Torque @ gears/1  "T_w_req (Nm)"
  Constant1/1 -> Subtract1/1
  Saturation/1 -> MaxSpinG1/1
  Saturation4/1 -> MaxWhlTorinG1/1
  Delay2/1 -> Subtract1/2, If Action Subsystem3/1(Selected Gear /dt), If Action Subsystem5/1(Selected Gear Ratio /dt), If Action Subsystem4/1(Selected Gear /dt), Saturation/1, Saturation4/1
  Subtract1/1 -> Scope5/1, GNo/1, To Workspace2/1
  v (m/s)/1 -> Scope6/1, If1/1
  If1/3 -> If Action Subsystem6/Action
  Constant2/1 -> If Action Subsystem6/1(In1)
  If Action Subsystem6/1(Out1) -> Merge1/3
  Merge1/1 -> Saturation2/1
  Avl Torque @ gears/1 -> Ceil/1
  Ceil/1 -> Saturation1/1
  Saturation Dynamic/1 -> Zero-Order Hold/1
  Constant3/1 -> Subtract/2
  Saturation1/1 -> Subtract/1
  Saturation2/1 -> Scope2/1, Saturation Dynamic/2
  Constant/1 -> Saturation Dynamic/3
  Subtract/1 -> Saturation Dynamic/1
  Zero-Order Hold/1 -> Delay2/1, Scope2/2, Clutch position definition/1(GNo)

== system Refined_Model_39/Environment/If Action Subsystem ==
  In1 : Inport
  Action Port : ActionPort  ActionPortLabel=if(u1 > 0)
  Out1 : Outport
  wires:
  In1/1 -> Out1/1

== system Refined_Model_39/Environment/If Action Subsystem1 ==
  In1 : Inport
  Action Port : ActionPort  ActionPortLabel=else
  Out1 : Outport
  wires:
  In1/1 -> Out1/1

== system Refined_Model_39/ICE Vehicle model/Axle ==
  T_g (Nm) : Inport
  W_g (rpm) : Inport  Port=2
  W_w_real (rpm) : Inport  Port=3
  Add4 : Sum  Inputs=-++
  Add5 : Sum
  Axle Loss Tables1 : Lookup_n-D  BreakpointsForDimension1=ALInpTor  BreakpointsForDimension2=ALInpSpeed  BreakpointsForDimension3=GNo  Table=ALTableVal  InterpMethod=Linear Lagrange  InternalRulePriority=Speed  RndMeth=Simplest  InputSameDT=on
      settings: InputPortMap=u0,u1
  Constant28 : Constant  Value=NoWhlFA
  Constant29 : Constant  Value=NoWhlRA
  Derivative6 : Derivative
  FDR4 : Gain  Gain=FDR
  FDR5 : Gain  Gain=1/FDR
  Gain12 : Gain  Gain=pi/30
  Gain26 : Gain  Gain=Jk
  Product10 : Product
  Scope : Scope
  Scope2 : Scope  NumInputPorts=2
  T_w (Nm) : Outport
  wires:
  Product10/1 -> Add4/3  "T_w_iner (Nm)"
  Derivative6/1 -> Gain26/1
  Add5/1 -> Product10/2
  Constant29/1 -> Add5/2
  Constant28/1 -> Add5/1
  FDR4/1 -> Add4/2
  FDR5/1 -> Scope2/2  "W_w (rpm)"
  Gain26/1 -> Product10/1
  Add4/1 -> T_w (Nm)/1, Scope/1  "T_w (Nm)"
  T_g (Nm)/1 -> Axle Loss Tables1/1, FDR4/1
  W_g (rpm)/1 -> FDR5/1
  W_w_real (rpm)/1 -> Gain12/1
  Axle Loss Tables1/1 -> Add4/1  "T_axl_loss (Nm)"
  Gain12/1 -> Scope2/1, Axle Loss Tables1/2, Derivative6/1

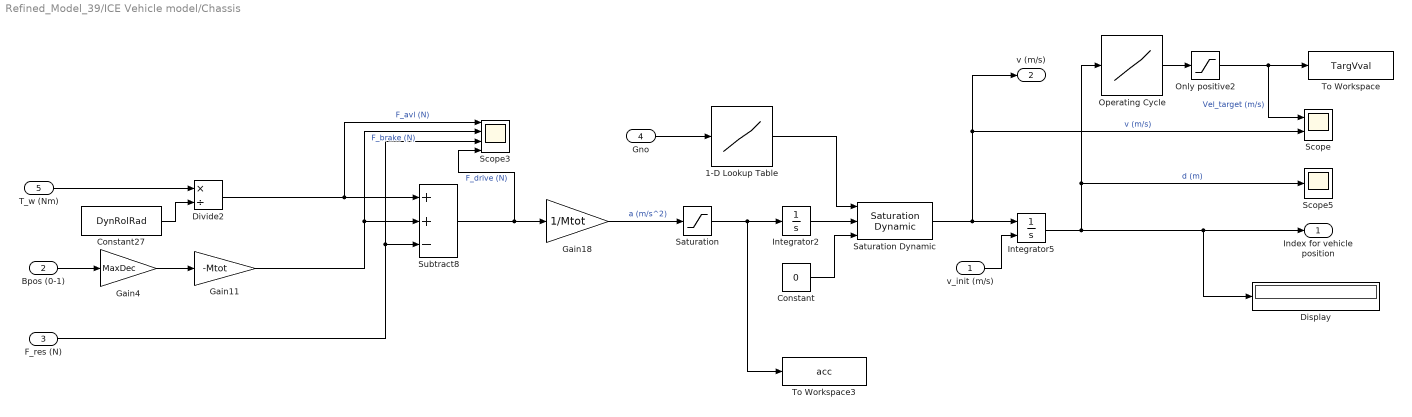
== system Refined_Model_39/ICE Vehicle model/Chassis ==
  v_init (m/s) : Inport
  Bpos (0-1) : Inport  Port=2
  F_res (N) : Inport  Port=3
  Gno : Inport  Port=4
  T_w (Nm) : Inport  Port=5
  1-D Lookup Table : Lookup_n-D  NumberOfTableDimensions=1  BreakpointsForDimension1=1:length(MaxSpinG)  Table=MaxSpinG  InternalRulePriority=Speed  RndMeth=Simplest  InputSameDT=on
  Constant : Constant  Value=0
  Constant27 : Constant  Value=DynRolRad
  Display : Display
  Divide2 : Product  Inputs=*/
  Gain11 : Gain  Gain=-Mtot
  Gain18 : Gain  Gain=1/Mtot
  Gain4 : Gain  Gain=MaxDec
  Integrator2 : Integrator  ContinuousStateAttributes='acceleration'
  Integrator5 : Integrator  InitialConditionSource=external  ContinuousStateAttributes='velocity'
  Only positive2 : Saturate  UpperLimit=inf  LowerLimit=0
  Operating Cycle : Lookup_n-D  NumberOfTableDimensions=1  BreakpointsForDimension1=Dist  BreakpointsForDimension2=G1Inprpm  Table=MaxSpeedProfile  InterpMethod=Linear Lagrange  InternalRulePriority=Speed  RndMeth=Simplest  InputSameDT=on
  Saturation : Saturate  UpperLimit=MaxAcc  LowerLimit=-(MaxDec)
  Saturation Dynamic : simulink/Discontinuities/Saturation Dynamic  OutMin=[]  OutMax=[]  OutDataTypeStr=Inherit: Same as second input  OutDataType=fixdt(1, 16)  OutScaling=2^-10  DoSatur=off
  Scope : Scope  NumInputPorts=2
  Scope3 : Scope  NumInputPorts=4
  Scope5 : Scope
  Subtract8 : Sum  Inputs=++-
  To Workspace : ToWorkspace  VariableName=TargVval  SaveFormat=Timeseries  SampleTime=-1
  To Workspace3 : ToWorkspace  VariableName=acc  SaveFormat=Timeseries  SampleTime=-1
  Index for vehicle position : Outport
  v (m/s) : Outport  Port=2
  wires:
  Constant27/1 -> Divide2/2
  Subtract8/1 -> Scope3/4, Gain18/1  "F_drive (N)"
  Divide2/1 -> Subtract8/1, Scope3/1  "F_avl (N)"
  Integrator5/1 -> Display/1, Index for vehicle position/1, Scope5/1, Operating Cycle/1  "d (m)"
  Integrator2/1 -> Saturation Dynamic/2
  T_w (Nm)/1 -> Divide2/1
  Gain11/1 -> Subtract8/2, Scope3/2  "F_brake (N)"
  Saturation Dynamic/1 -> Scope/2, v (m/s)/1, Integrator5/1  "v (m/s)"
  v_init (m/s)/1 -> Integrator5/2
  Operating Cycle/1 -> Only positive2/1
  Gain18/1 -> Saturation/1  "a (m/s^2)"
  Bpos (0-1)/1 -> Gain4/1
  Gain4/1 -> Gain11/1
  F_res (N)/1 -> Subtract8/3, Scope3/3
  Saturation/1 -> Integrator2/1, To Workspace3/1
  Only positive2/1 -> Scope/1, To Workspace/1  "Vel_target (m/s)"
  Constant/1 -> Saturation Dynamic/3
  Gno/1 -> 1-D Lookup Table/1
  1-D Lookup Table/1 -> Saturation Dynamic/1

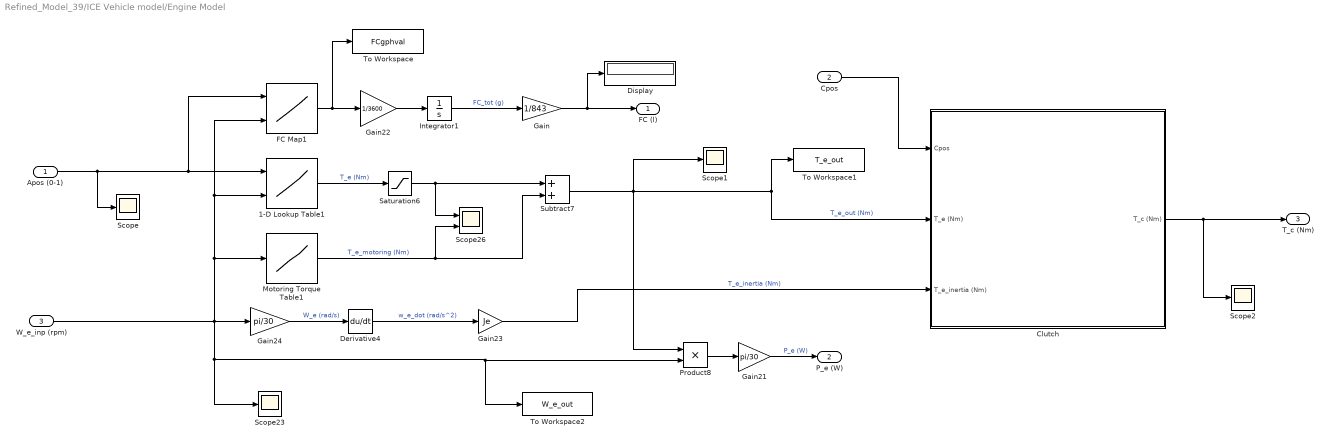
== system Refined_Model_39/ICE Vehicle model/Engine Model ==
  Apos (0-1) : Inport
  Cpos : Inport  Port=2
  W_e_inp (rpm) : Inport  Port=3
  1-D Lookup Table1 : Lookup_n-D  BreakpointsForDimension1=ThrotPos  BreakpointsForDimension2=RpmBrkPnt  Table=ThrotTableVal  InternalRulePriority=Speed  RndMeth=Simplest  InputSameDT=on
      settings: InputPortMap=u0,u1
  Clutch : Subsystem
  Derivative4 : Derivative
  Display : Display
  FC Map1 : Lookup_n-D  BreakpointsForDimension1=ThrotPos  BreakpointsForDimension2=RpmBrkPnt  Table=FCTableVal  InternalRulePriority=Speed  RndMeth=Simplest  InputSameDT=on
      settings: InputPortMap=u0,u1
  Gain : Gain  Gain=1/843
  Gain21 : Gain  Gain=pi/30
  Gain22 : Gain  Gain=1/3600
  Gain23 : Gain  Gain=Je
  Gain24 : Gain  Gain=pi/30
  Integrator1 : Integrator
  Motoring Torque Table1 : Lookup_n-D  NumberOfTableDimensions=1  BreakpointsForDimension1=EngineRpm  BreakpointsForDimension2=G1Inprpm  Table=MotoringTor  InterpMethod=Linear Lagrange  InternalRulePriority=Speed  RndMeth=Simplest  InputSameDT=on
  Product8 : Product
  Saturation6 : Saturate  UpperLimit=max(ThrotTableVal, [], 'all')  LowerLimit=0
  Scope{,1..2,23} (4 alike) : Scope
  Scope26 : Scope  NumInputPorts=2
  Subtract7 : Sum
  To Workspace : ToWorkspace  VariableName=FCgphval  SaveFormat=Timeseries  SampleTime=-1
  To Workspace1 : ToWorkspace  VariableName=T_e_out  SaveFormat=Timeseries  SampleTime=-1
  To Workspace2 : ToWorkspace  VariableName=W_e_out  SaveFormat=Timeseries  SampleTime=-1
  FC (l) : Outport
  P_e (W) : Outport  Port=2
  T_c (Nm) : Outport  Port=3
  wires:
  Motoring Torque Table1/1 -> Subtract7/2, Scope26/2  "T_e_motoring (Nm)"
  Integrator1/1 -> Gain/1  "FC_tot (g)"
  Derivative4/1 -> Gain23/1  "w_e_dot (rad/s^2)"
  W_e_inp (rpm)/1 -> Scope23/1, To Workspace2/1, Product8/2, FC Map1/2, 1-D Lookup Table1/2, Motoring Torque Table1/1, Gain24/1
  Product8/1 -> Gain21/1
  Apos (0-1)/1 -> FC Map1/1, 1-D Lookup Table1/1, Scope/1
  1-D Lookup Table1/1 -> Saturation6/1  "T_e (Nm)"
  Gain24/1 -> Derivative4/1  "W_e (rad/s)"
  Gain23/1 -> Clutch/3(T_e_inertia (Nm))  "T_e_inertia (Nm)"
  Gain21/1 -> P_e (W)/1  "P_e (W)"
  Gain22/1 -> Integrator1/1
  Subtract7/1 -> To Workspace1/1, Clutch/2(T_e (Nm)), Scope1/1, Product8/1  "T_e_out (Nm)"
  FC Map1/1 -> To Workspace/1, Gain22/1
  Saturation6/1 -> Scope26/1, Subtract7/1
  Clutch/1(T_c (Nm)) -> Scope2/1, T_c (Nm)/1
  Cpos/1 -> Clutch/1(Cpos)
  Gain/1 -> Display/1, FC (l)/1

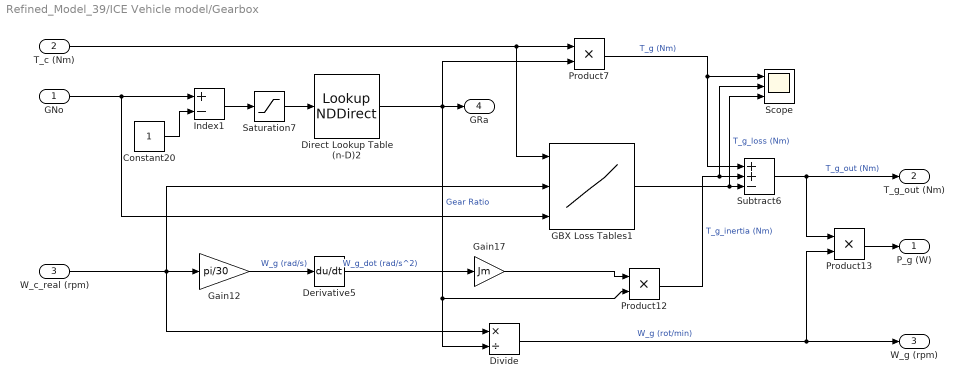
== system Refined_Model_39/ICE Vehicle model/Gearbox ==
  GNo : Inport
  T_c (Nm) : Inport  Port=2
  W_c_real (rpm) : Inport  Port=3
  Constant20 : Constant
  Derivative5 : Derivative
  Direct Lookup Table (n-D)2 : LookupNDDirect  NumberOfTableDimensions=1  Table=GRa
  Divide : Product  Inputs=*/
  GBX Loss Tables1 : Lookup_n-D  NumberOfTableDimensions=3  BreakpointsForDimension1=GInpTor  BreakpointsForDimension2=GInprpm  BreakpointsForDimension3=GNo  Table=GTorLoss  InterpMethod=Linear Lagrange  InternalRulePriority=Speed  RndMeth=Simplest  InputSameDT=on
      settings: InputPortMap=u0,u1,u2
  Gain12 : Gain  Gain=pi/30
  Gain17 : Gain  Gain=Jm
  Index1 : Sum  Inputs=+-
  Product12 : Product
  Product13 : Product
  Product7 : Product
  Saturation7 : Saturate  UpperLimit=inf  LowerLimit=0
  Scope : Scope  NumInputPorts=3
  Subtract6 : Sum  Inputs=++-
  P_g (W) : Outport
  T_g_out (Nm) : Outport  Port=2
  W_g (rpm) : Outport  Port=3
  GRa : Outport  Port=4
  wires:
  Product12/1 -> Scope/2, Subtract6/2  "T_g_inertia (Nm)"
  GNo/1 -> Index1/1, GBX Loss Tables1/3
  Gain17/1 -> Product12/1
  T_c (Nm)/1 -> GBX Loss Tables1/1, Product7/1
  Product7/1 -> Subtract6/1, Scope/1  "T_g (Nm)"
  Divide/1 -> W_g (rpm)/1, Product13/2  "W_g (rot/min)"
  Subtract6/1 -> T_g_out (Nm)/1, Product13/1  "T_g_out (Nm)"
  Derivative5/1 -> Gain17/1  "W_g_dot (rad/s^2)"
  Direct Lookup Table (n-D)2/1 -> GRa/1, Product7/2, Product12/2, Divide/2  "Gear Ratio"
  Saturation7/1 -> Direct Lookup Table (n-D)2/1
  Gain12/1 -> Derivative5/1  "W_g (rad/s)"
  Constant20/1 -> Index1/2
  GBX Loss Tables1/1 -> Scope/3, Subtract6/3  "T_g_loss (Nm)"
  Index1/1 -> Saturation7/1
  Product13/1 -> P_g (W)/1
  W_c_real (rpm)/1 -> Gain12/1, Divide/1, GBX Loss Tables1/2

== system Refined_Model_39/Driver Model/Acc//Dec Control/Driving state ==
  v (m/s) : Inport
  d (m) : Inport  Port=2
  Constant : Constant  Value=0
  Constant2 : Constant
  Constant3 : Constant  Value=0
  Delay : Delay  DelayLength=1
  Idling at stop point : If  NumInputs=2  IfExpression=u1 == 0 & u2 > 0
  If Action Subsystem : Subsystem  TreatAsAtomicUnit=on
  If Action Subsystem1 : Subsystem  TreatAsAtomicUnit=on
  Merge : Merge
  Stop duration1 : Subsystem
  Stop idling after stop duration : Switch  Criteria=u2 > Threshold
  Trip complete : Subsystem
  Vehicle temporary stop timer : VariableTransportDelay  VariableDelayType=Variable transport delay  MaximumDelay=10
  Engine_Idle : Outport
  wires:
  Constant2/1 -> If Action Subsystem/1(In1)
  If Action Subsystem/1(Out1) -> Merge/1
  Merge/1 -> Delay/1
  Idling at stop point/1 -> If Action Subsystem/Action
  Constant3/1 -> If Action Subsystem1/1(In1)
  Idling at stop point/2 -> If Action Subsystem1/Action
  If Action Subsystem1/1(Out1) -> Merge/2
  v (m/s)/1 -> Idling at stop point/1
  d (m)/1 -> Trip complete/1(d (m)), Stop duration1/1(d (m)), Idling at stop point/2
  Constant/1 -> Stop idling after stop duration/1
  Stop duration1/1(Stop_t (s)) -> Vehicle temporary stop timer/2  "Stop_t (s)"
  Vehicle temporary stop timer/1 -> Stop idling after stop duration/2
  Delay/1 -> Vehicle temporary stop timer/1, Stop idling after stop duration/3  "Engine_Idle"
  Stop idling after stop duration/1 -> Engine_Idle/1

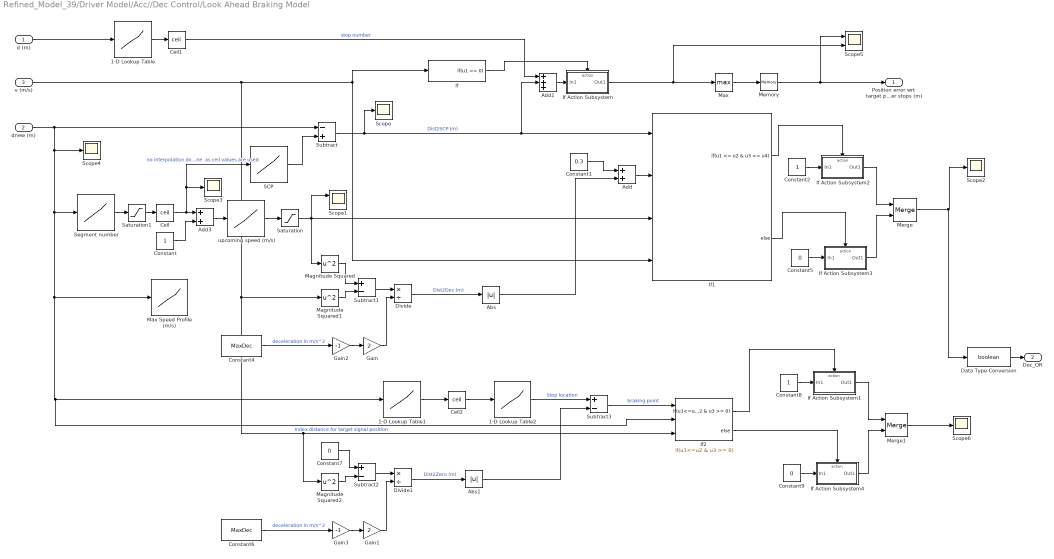
== system Refined_Model_39/Driver Model/Acc//Dec Control/Look Ahead Braking Model ==
  d (m) : Inport
  dnew (m) : Inport  Port=2
  v (m/s) : Inport  Port=3
  1-D Lookup Table : Lookup_n-D  NumberOfTableDimensions=1  BreakpointsForDimension1=Stoptimes(:,1)  Table=1:length(Stoptimes)  InternalRulePriority=Speed  RndMeth=Simplest  InputSameDT=on
  1-D Lookup Table1 : Lookup_n-D  NumberOfTableDimensions=1  BreakpointsForDimension1=Stoptimes(:,1)  Table=1:length(Stoptimes)  InternalRulePriority=Speed  RndMeth=Simplest  InputSameDT=on
  1-D Lookup Table2 : Lookup_n-D  NumberOfTableDimensions=1  BreakpointsForDimension1=1:length(Stoptimes)  Table=Stoptimes(:,1)  InternalRulePriority=Speed  RndMeth=Simplest  InputSameDT=on
  Abs : Abs
  Abs1 : Abs
  Add : Sum
  Add1 : Sum  Inputs=+++
  Add3 : Sum
  Ceil : Rounding  Operator=ceil
  Ceil1 : Rounding  Operator=ceil
  Ceil2 : Rounding  Operator=ceil
  Constant : Constant
  Constant1 : Constant  Value=0.3
  Constant2 : Constant
  Constant4 : Constant  Value=MaxDec
  Constant5 : Constant  Value=0
  Constant6 : Constant  Value=MaxDec
  Constant7 : Constant  Value=0
  Constant8 : Constant
  Constant9 : Constant  Value=0
  Data Type Conversion : DataTypeConversion  OutDataTypeStr=boolean
  Divide : Product  Inputs=*/
  Divide1 : Product  Inputs=*/
  Gain : Gain  Gain=2
  Gain1 : Gain  Gain=2
  Gain2 : Gain  Gain=-1
  Gain3 : Gain  Gain=-1
  If : If  IfExpression=u1 == 0  ShowElse=off
  If Action Subsystem : Subsystem  TreatAsAtomicUnit=on
  If Action Subsystem1 : Subsystem  TreatAsAtomicUnit=on
  If Action Subsystem2 : Subsystem  TreatAsAtomicUnit=on
  If Action Subsystem3 : Subsystem  TreatAsAtomicUnit=on
  If Action Subsystem4 : Subsystem  TreatAsAtomicUnit=on
  If1 : If  NumInputs=4  IfExpression=u1 <= u2 & u3 <= u4
  If2 : If  NumInputs=3  IfExpression=u1<=u2 & u3 >= 0
  Magnitude Squared : Math  Operator=square  SaturateOnIntegerOverflow=on
  Magnitude Squared1 : Math  Operator=square  SaturateOnIntegerOverflow=on
  Magnitude Squared2 : Math  Operator=square  SaturateOnIntegerOverflow=on
  Max : MinMax  Function=max
  Max Speed Profile (m/s) : Lookup_n-D  NumberOfTableDimensions=1  BreakpointsForDimension1=Dist  BreakpointsForDimension2=G1Inprpm  Table=MaxSpeedProfile  InterpMethod=Linear Lagrange  InternalRulePriority=Speed  RndMeth=Simplest  InputSameDT=on
  Memory : Memory
  Merge : Merge
  Merge1 : Merge
  SCP : Lookup_n-D  NumberOfTableDimensions=1  BreakpointsForDimension1=SegNo  BreakpointsForDimension2=G1Inprpm  Table=CovDist  InterpMethod=Linear Lagrange  InternalRulePriority=Speed  RndMeth=Simplest  InputSameDT=on
  Saturation : Saturate  UpperLimit=inf  LowerLimit=0
  Saturation1 : Saturate  UpperLimit=inf  LowerLimit=0
  Scope{,2..4,6} (5 alike) : Scope
  Scope1 : Scope  NumInputPorts=2
  Scope5 : Scope  NumInputPorts=2
  Segment number : Lookup_n-D  NumberOfTableDimensions=1  BreakpointsForDimension1=CovDist  BreakpointsForDimension2=G1Inprpm  Table=SegNo  InterpMethod=Linear Lagrange  InternalRulePriority=Speed  RndMeth=Simplest  InputSameDT=on
  Subtract : Sum  Inputs=-+
  Subtract1 : Sum  Inputs=+-
  Subtract2 : Sum  Inputs=+-
  Subtract3 : Sum  Inputs=+-
  upcoming speed (m/s) : Lookup_n-D  NumberOfTableDimensions=1  BreakpointsForDimension1=SegNo  BreakpointsForDimension2=G1Inprpm  Table=SegSPLatinmps  InterpMethod=Linear Lagrange  InternalRulePriority=Speed  RndMeth=Simplest  InputSameDT=on
  Position error wrt target position after stops (m) : Outport
  Dec_OR : Outport  Port=2
  wires:
  Add3/1 -> upcoming speed (m/s)/1
  Ceil/1 -> Add3/1, Scope3/1, SCP/1  "no interpolation done  as ceil values are used"
  SCP/1 -> Subtract/2
  Constant/1 -> Add3/2
  Subtract/1 -> If1/1, Add1/2, Scope/1  "Dist2SCP (m)"
  Segment number/1 -> Saturation1/1
  Magnitude Squared/1 -> Subtract1/1
  Constant4/1 -> Gain2/1  "deceleration in m/s^2"
  Divide/1 -> Abs/1  "Dist2Dec (m)"
  Constant2/1 -> If Action Subsystem2/1(In1)
  If1/1 -> If Action Subsystem2/Action
  If Action Subsystem2/1(Out1) -> Merge/1
  Magnitude Squared1/1 -> Subtract1/2
  Data Type Conversion/1 -> Dec_OR/1
  dnew (m)/1 -> Subtract/1, Scope4/1, Segment number/1, If2/2, 1-D Lookup Table1/1, Max Speed Profile (m/s)/1  "Index distance for target signal position"
  Subtract1/1 -> Divide/1
  Gain2/1 -> Gain/1
  Gain/1 -> Divide/2
  upcoming speed (m/s)/1 -> Saturation/1
  Saturation1/1 -> Ceil/1
  Merge/1 -> Data Type Conversion/1, Scope2/1
  Constant5/1 -> If Action Subsystem3/1(In1)
  If Action Subsystem3/1(Out1) -> Merge/2
  If1/2 -> If Action Subsystem3/Action
  If/1 -> If Action Subsystem/Action
  Add1/1 -> If Action Subsystem/1(In1)
  Max/1 -> Memory/1
  1-D Lookup Table/1 -> Ceil1/1
  Ceil1/1 -> Add1/1  "stop number"
  Abs/1 -> Add/2
  1-D Lookup Table1/1 -> Ceil2/1
  Ceil2/1 -> 1-D Lookup Table2/1
  Constant6/1 -> Gain3/1  "deceleration in m/s^2"
  Gain1/1 -> Divide1/2
  Constant7/1 -> Subtract2/1
  Divide1/1 -> Abs1/1  "Dist2Zero (m)"
  Subtract2/1 -> Divide1/1
  Gain3/1 -> Gain1/1
  Magnitude Squared2/1 -> Subtract2/2
  1-D Lookup Table2/1 -> Subtract3/1  "Stop location"
  Subtract3/1 -> If2/1  "braking point"
  If Action Subsystem4/1(Out1) -> Merge1/2
  If2/2 -> If Action Subsystem4/Action
  Constant8/1 -> If Action Subsystem1/1(In1)
  Constant9/1 -> If Action Subsystem4/1(In1)
  Merge1/1 -> Scope6/1
  If Action Subsystem1/1(Out1) -> Merge1/1
  If2/1 -> If Action Subsystem1/Action
  Abs1/1 -> Subtract3/2
  Add/1 -> If1/2
  Constant1/1 -> Add/1
  If Action Subsystem/1(Out1) -> Scope5/2, Max/1
  Memory/1 -> Scope5/1, Position error wrt target position after stops (m)/1
  d (m)/1 -> 1-D Lookup Table/1
  v (m/s)/1 -> Magnitude Squared2/1, If2/3, Magnitude Squared1/1, If/1, If1/4
  Saturation/1 -> If1/3, Scope1/1, Magnitude Squared/1

== system Refined_Model_39/Driver Model/Driver Throttle Mapping ICE/Idling// Apos = 0 ==
  Apos(m/s^2) : Inport
  Constant : Constant
  Constant2 : Constant  Value=0
  Idling : If  IfExpression=u1 == 0
  If Action Subsystem : Subsystem  TreatAsAtomicUnit=on
  If Action Subsystem1 : Subsystem  TreatAsAtomicUnit=on
  Merge : Merge
  Azero : Outport
  wires:
  Constant2/1 -> If Action Subsystem1/1(In1)
  Idling/1 -> If Action Subsystem/Action
  Merge/1 -> Azero/1
  If Action Subsystem1/1(Out1) -> Merge/1
  Constant/1 -> If Action Subsystem/1(In1)
  Apos(m/s^2)/1 -> Idling/1
  Idling/2 -> If Action Subsystem1/Action
  If Action Subsystem/1(Out1) -> Merge/2

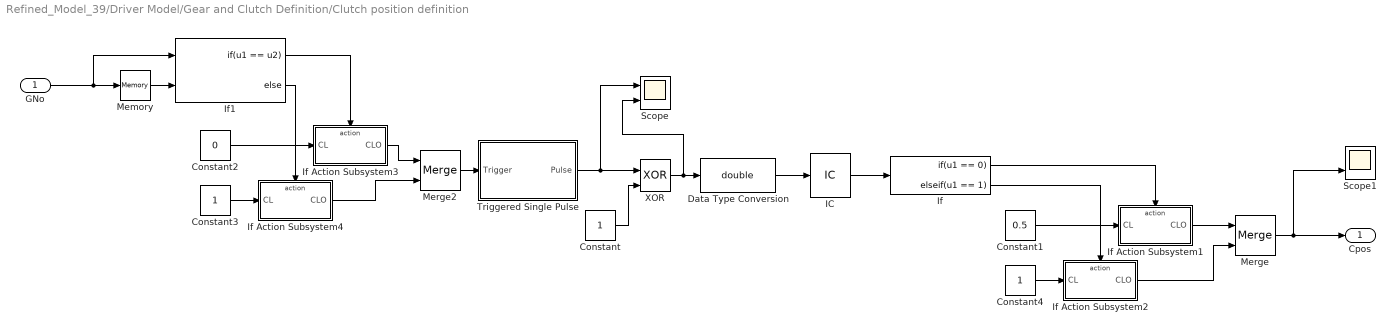
== system Refined_Model_39/Driver Model/Gear and Clutch Definition/Clutch position definition ==
  GNo : Inport
  Constant : Constant
  Constant1 : Constant  Value=0.5
  Constant2 : Constant  Value=0
  Constant3 : Constant
  Constant4 : Constant
  Data Type Conversion : DataTypeConversion  OutDataTypeStr=double
  IC : InitialCondition  Value=0
  If : If  IfExpression=u1 == 0  ElseIfExpressions=u1 == 1  ShowElse=off
  If Action Subsystem1 : Subsystem  TreatAsAtomicUnit=on
  If Action Subsystem2 : Subsystem  TreatAsAtomicUnit=on
  If Action Subsystem3 : Subsystem  TreatAsAtomicUnit=on
  If Action Subsystem4 : Subsystem  TreatAsAtomicUnit=on
  If1 : If  NumInputs=2  IfExpression=u1 == u2
  Memory : Memory
  Merge : Merge
  Merge2 : Merge
  Scope : Scope  NumInputPorts=2
  Scope1 : Scope  NumInputPorts=2
  Triggered Single Pulse : Subsystem  TreatAsAtomicUnit=on  mask(single pulse generation){p_wid=4}
      mask prompts: p_wid "pulse width (number of samples)"
      mask help: This block generate a single pulse whenever a trigger happen. The pulse width must specified as a number of samples. for example if your sampling time is 0.1s and you want 3s pulse , then you should enter 30 as a pulse width.
      mask Display:
      | plot([0],[0])
      | plot([11],[0])
      | plot([5],[0.5])
      | plot([4 5 5 6 6 7],[0 0 0.25 0.25 0 0])
      | plot([5],[-0.3])
      | 
      | port_label('output', 1, 'Pulse')
      | port_label('input', 1, 'Trigger')
  XOR : Logic  Operator=XOR  IconShape=distinctive  AllPortsSameDT=off  OutDataTypeStr=boolean
  Cpos : Outport
  wires:
  If1/1 -> If Action Subsystem3/Action
  If Action Subsystem3/1(CLO) -> Merge2/1
  Memory/1 -> If1/2
  Constant2/1 -> If Action Subsystem3/1(CL)
  Constant3/1 -> If Action Subsystem4/1(CL)
  GNo/1 -> Memory/1, If1/1
  If1/2 -> If Action Subsystem4/Action
  If Action Subsystem4/1(CLO) -> Merge2/2
  Merge2/1 -> Triggered Single Pulse/1(Trigger)
  Triggered Single Pulse/1(Pulse) -> Scope/1, XOR/1
  Constant/1 -> XOR/2
  XOR/1 -> Scope/2, Data Type Conversion/1
  Data Type Conversion/1 -> IC/1
  IC/1 -> If/1
  Constant4/1 -> If Action Subsystem2/1(CL)
  Constant1/1 -> If Action Subsystem1/1(CL)
  If Action Subsystem2/1(CLO) -> Merge/2
  If/2 -> If Action Subsystem2/Action
  If/1 -> If Action Subsystem1/Action
  If Action Subsystem1/1(CLO) -> Merge/1
  Merge/1 -> Scope1/2, Cpos/1

== system Refined_Model_39/Driver Model/Gear and Clutch Definition/If Action Subsystem3 ==
  Selected Gear /dt : Inport
  Action Port : ActionPort  ActionPortLabel=if(u1 >= u2)
  Add : Sum
  Constant : Constant
  Increased gear : Outport
  wires:
  Selected Gear /dt/1 -> Add/1
  Add/1 -> Increased gear/1
  Constant/1 -> Add/2

== system Refined_Model_39/Driver Model/Gear and Clutch Definition/If Action Subsystem4 ==
  Selected Gear /dt : Inport
  Action Port : ActionPort  ActionPortLabel=elseif(u3 >= u4)
  Constant : Constant
  Subtract : Sum  Inputs=+-
  Decreased gear : Outport
  wires:
  Constant/1 -> Subtract/2
  Subtract/1 -> Decreased gear/1
  Selected Gear /dt/1 -> Subtract/1

== system Refined_Model_39/Driver Model/Gear and Clutch Definition/If Action Subsystem5 ==
  Selected Gear Ratio /dt : Inport
  Action Port : ActionPort  ActionPortLabel=else
  Out1 : Outport
  wires:
  Selected Gear Ratio /dt/1 -> Out1/1

== system Refined_Model_39/Driver Model/Gear and Clutch Definition/If Action Subsystem6 ==
  In1 : Inport
  Action Port : ActionPort  ActionPortLabel=elseif(u1 == 0)
  Out1 : Outport
  wires:
  In1/1 -> Out1/1

== system Refined_Model_39/ICE Vehicle model/Engine Model/Clutch ==
  Cpos : Inport
  T_e (Nm) : Inport  Port=2
  T_e_inertia (Nm) : Inport  Port=3
  Add : Sum
  Clutch value1 : Product
  Gain20 : Gain  Gain=etaClutch
  Saturation2 : Saturate  UpperLimit=inf  LowerLimit=0
  Scope : Scope
  Scope1 : Scope  NumInputPorts=2
  T_c (Nm) : Outport
  wires:
  Cpos/1 -> Clutch value1/1
  Clutch value1/1 -> Gain20/1
  Gain20/1 -> Saturation2/1  "T_c (Nm)"
  T_e_inertia (Nm)/1 -> Add/2, Scope1/2
  T_e (Nm)/1 -> Add/1
  Saturation2/1 -> Scope/1, T_c (Nm)/1
  Add/1 -> Scope1/1, Clutch value1/2

== system Refined_Model_39/Driver Model/Acc//Dec Control/Driving state/If Action Subsystem ==
  In1 : Inport
  Action Port : ActionPort  ActionPortLabel=if(u1 == 0 & u2 > 0)
  Out1 : Outport
  wires:
  In1/1 -> Out1/1

== system Refined_Model_39/Driver Model/Acc//Dec Control/Driving state/If Action Subsystem1 ==
  In1 : Inport
  Action Port : ActionPort  ActionPortLabel=else
  Out1 : Outport
  wires:
  In1/1 -> Out1/1

== system Refined_Model_39/Driver Model/Acc//Dec Control/Driving state/Stop duration1 ==
  d (m) : Inport
  1-D Lookup Table : Lookup_n-D  NumberOfTableDimensions=1  BreakpointsForDimension1=Stoptimes(:,1)  Table=1:length(Stoptimes)  InternalRulePriority=Speed  RndMeth=Simplest  InputSameDT=on
  Ceil : Rounding  Operator=ceil
  Constant2 : Constant
  Direct Lookup Table (n-D) : LookupNDDirect  NumberOfTableDimensions=1  Table=Stoptimes(:,2)
  Scope : Scope
  Subtract1 : Sum  Inputs=+-
  Stop_t (s) : Outport
  wires:
  1-D Lookup Table/1 -> Ceil/1
  d (m)/1 -> 1-D Lookup Table/1
  Subtract1/1 -> Direct Lookup Table (n-D)/1
  Direct Lookup Table (n-D)/1 -> Stop_t (s)/1, Scope/1  "Stop time (s)"
  Ceil/1 -> Subtract1/1
  Constant2/1 -> Subtract1/2

== system Refined_Model_39/Driver Model/Acc//Dec Control/Driving state/Trip complete ==
  d (m) : Inport
  Constant1 : Constant  Value=NoSteps
  Constant2 : Constant
  Delay : Delay  DelayLength=1
  Derivative : Derivative
  If : If  NumInputs=3  IfExpression=u1 >= u2 & u3 ==0  ShowElse=off
  If Action Subsystem : Subsystem  TreatAsAtomicUnit=on
  Max : MinMax  Function=max
  Stop Simulation : Stop
  wires:
  Constant1/1 -> If/2
  Constant2/1 -> If Action Subsystem/1(In1)
  If/1 -> If Action Subsystem/Action
  If Action Subsystem/1(Out1) -> Delay/1
  d (m)/1 -> Max/1, Derivative/1
  Delay/1 -> Stop Simulation/1
  Derivative/1 -> If/3  "v (m/s)"
  Max/1 -> If/1

== system Refined_Model_39/Driver Model/Acc//Dec Control/Look Ahead Braking Model/If Action Subsystem ==
  In1 : Inport
  Action Port : ActionPort  ActionPortLabel=if(u1 == 0)
  Out1 : Outport
  wires:
  In1/1 -> Out1/1

== system Refined_Model_39/Driver Model/Acc//Dec Control/Look Ahead Braking Model/If Action Subsystem1 ==
  In1 : Inport
  Action Port : ActionPort  ActionPortLabel=if(u1<=u2 & u3 >= 0)
  Out1 : Outport
  wires:
  In1/1 -> Out1/1

== system Refined_Model_39/Driver Model/Acc//Dec Control/Look Ahead Braking Model/If Action Subsystem2 ==
  In1 : Inport
  Action Port : ActionPort  ActionPortLabel=if(u1 <= u2 & u3 <= u4)
  Out1 : Outport
  wires:
  In1/1 -> Out1/1

== system Refined_Model_39/Driver Model/Acc//Dec Control/Look Ahead Braking Model/If Action Subsystem3 ==
  In1 : Inport
  Action Port : ActionPort  ActionPortLabel=else
  Out1 : Outport
  wires:
  In1/1 -> Out1/1

== system Refined_Model_39/Driver Model/Acc//Dec Control/Look Ahead Braking Model/If Action Subsystem4 ==
  In1 : Inport
  Action Port : ActionPort  ActionPortLabel=else
  Out1 : Outport
  wires:
  In1/1 -> Out1/1

== system Refined_Model_39/Driver Model/Driver Throttle Mapping ICE/Idling// Apos = 0/If Action Subsystem ==
  In1 : Inport
  Action Port : ActionPort  ActionPortLabel=if(u1 == 0)
  Out1 : Outport
  wires:
  In1/1 -> Out1/1

== system Refined_Model_39/Driver Model/Driver Throttle Mapping ICE/Idling// Apos = 0/If Action Subsystem1 ==
  In1 : Inport
  Action Port : ActionPort  ActionPortLabel=else
  Out1 : Outport
  wires:
  In1/1 -> Out1/1

== system Refined_Model_39/Driver Model/Gear and Clutch Definition/Clutch position definition/If Action Subsystem1 ==
  CL : Inport
  Action Port : ActionPort  ActionPortLabel=if(u1 == 0)
  CLO : Outport
  wires:
  CL/1 -> CLO/1

== system Refined_Model_39/Driver Model/Gear and Clutch Definition/Clutch position definition/If Action Subsystem2 ==
  CL : Inport
  Action Port : ActionPort  ActionPortLabel=elseif(u1 == 1)
  CLO : Outport
  wires:
  CL/1 -> CLO/1

== system Refined_Model_39/Driver Model/Gear and Clutch Definition/Clutch position definition/If Action Subsystem3 ==
  CL : Inport
  Action Port : ActionPort  ActionPortLabel=if(u1 == u2)
  CLO : Outport
  wires:
  CL/1 -> CLO/1

== system Refined_Model_39/Driver Model/Gear and Clutch Definition/Clutch position definition/If Action Subsystem4 ==
  CL : Inport
  Action Port : ActionPort  ActionPortLabel=else
  CLO : Outport
  wires:
  CL/1 -> CLO/1
